simulink subsystem "CheckOutput_Bypass"  (R2021a)
settings: Solver=VariableStepAuto  StartTime=0.0  StopTime=10.0  RelTol=1e-3
undefined symbols (not defined in the file): ErrVarCheckOut
settings Model: Creator=zurnmar  LastModifiedBy=zurnmar

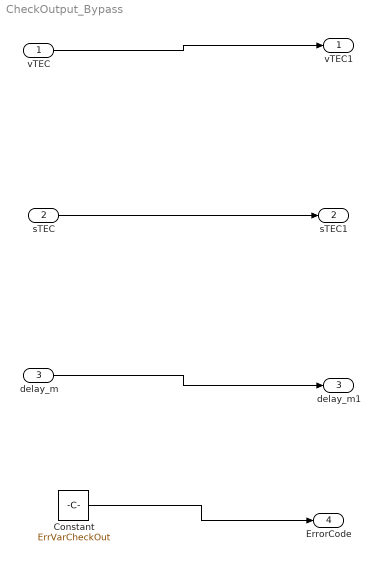
== system CheckOutput_Bypass ==
  vTEC : Inport
  sTEC : Inport  Port=2
  delay_m : Inport  Port=3
  Constant : Constant  Value=ErrVarCheckOut  OutDataTypeStr=uint16
  vTEC1 : Outport
  sTEC1 : Outport  Port=2
  delay_m1 : Outport  Port=3
  ErrorCode : Outport  Port=4
  wires:
  vTEC/1 -> vTEC1/1
  sTEC/1 -> sTEC1/1
  delay_m/1 -> delay_m1/1
  Constant/1 -> ErrorCode/1
